simulink model "zoomLensWithoutLookupTbl"  (Simulink 6.1)
settings: Solver=ode45  StartTime=0.0  StopTime=3  RelTol=1e-3
settings Model: LastModifiedBy=Big E
settings DebuggingCC: SolverPrmCheckMsg=warning

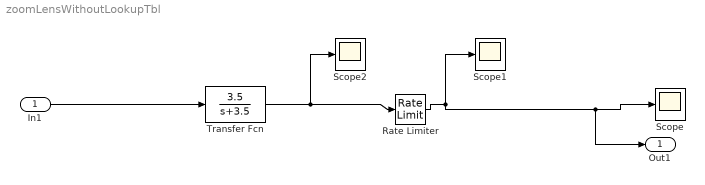
== system zoomLensWithoutLookupTbl ==
  In1 : Inport  Port=1  LatchInput=off
  Rate Limiter : RateLimiter  SampleTimeMode=inherited
  Scope : Scope
      settings: YMin=0  YMax=750
  Scope1 : Scope
      settings: YMin=0  YMax=750
  Scope2 : Scope
      settings: YMin=0  YMax=750  SaveName=ScopeData2
  Transfer Fcn : TransferFcn  Numerator=[3.5]  Denominator=[1 3.5]
  Out1 : Outport
  wires:
  Transfer Fcn/1 -> Rate Limiter/1, Scope2/1
  Rate Limiter/1 -> Scope1/1, Scope/1, Out1/1
  In1/1 -> Transfer Fcn/1
